simulink model "Model_Following_Approach"  (Simulink 7.5)
settings: Solver=ode45  StartTime=0.0  StopTime=10.0  RelTol=1e-3
values from neighbouring files (symbols this model uses):
  A_r = [ -1  -1   0   0 ... (first row only)    [main_c.m]    (also in main_elca.m; main_elca_nonsquare.m; main_elca_siso.m; main_elca_siso_conference.m)
  B_r = [ 1  0 ... (first row only)    [main_c.m]    (also in main_elca.m; main_elca_nonsquare.m = B_r(:,1:m); main_elca_siso.m = B_r(:,1:m); main_elca_siso_conference.m = [ 1)
  C_r = [ 1  0  0  0 ... (first row only)    [main_c.m]    (also in main_elca.m; main_elca_nonsquare.m = C_r(1:p,:); main_elca_siso.m = C_r(1:p,:); main_elca_siso_conference.m = [ 1  0  0  0])
  D_r = zeros(pr,mr)    [main_c.m]    (also in main_elca.m; main_elca_nonsquare.m; main_elca_siso.m; main_elca_siso_conference.m)
  Er = -inv(Rr)*B_r'*inv( A_r - B_r*Kr )'*C_r'*Qr    [main_c.m]    (also in main_elca.m; main_elca_nonsquare.m; main_elca_siso.m; main_elca_siso_conference.m)
  x_r = X_r'    [main_c.m]    (also in main_elca.m; main_elca_nonsquare.m; main_elca_siso.m; main_elca_siso_conference.m)
undefined symbols (not defined in the file or in its folder): Kr
settings Model: Creator=koni  LastModifiedBy=koni

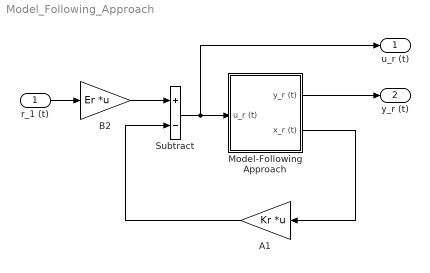
== system Model_Following_Approach ==
  r_1 (t) : Inport  PortDimensions=pr
  " Model-Following Approach" : Subsystem
  A1 : Gain  Gain=Kr  Multiplication=Matrix(K*u)  ParameterDataType=fixdt(1, 16)  ParameterScaling=2^0  OutDataType=fixdt(1, 16)  OutScaling=2^0
  B2 : Gain  Gain=Er  Multiplication=Matrix(K*u)  ParameterDataType=fixdt(1, 16)  ParameterScaling=2^0  OutDataType=fixdt(1, 16)  OutScaling=2^0
  Subtract : Sum  Inputs=+-  OutDataType=fixdt(1, 16)  OutScaling=2^-10
  u_r (t) : Outport  PortDimensions=mr  OutDataType=fixdt(1, 16)  OutScaling=2^0
  y_r (t) : Outport  Port=2  PortDimensions=pr  OutDataType=fixdt(1, 16)  OutScaling=2^0
  wires:
  " Model-Following Approach"/1(y_r (t)) -> y_r (t)/1
  Subtract/1 -> " Model-Following Approach"/1(u_r (t)), u_r (t)/1
  B2/1 -> Subtract/1
  r_1 (t)/1 -> B2/1
  " Model-Following Approach"/2(x_r (t)) -> A1/1
  A1/1 -> Subtract/2

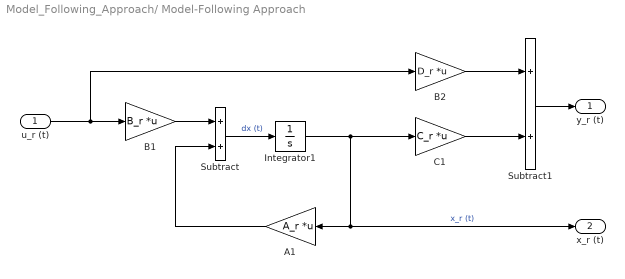
== system Model_Following_Approach/ Model-Following Approach ==
  u_r (t) : Inport  PortDimensions=mr
  A1 : Gain  Gain=A_r  Multiplication=Matrix(K*u)  ParameterDataType=fixdt(1, 16)  ParameterScaling=2^0  OutDataType=fixdt(1, 16)  OutScaling=2^0
  B1 : Gain  Gain=B_r  Multiplication=Matrix(K*u)  ParameterDataType=fixdt(1, 16)  ParameterScaling=2^0  OutDataType=fixdt(1, 16)  OutScaling=2^0
  B2 : Gain  Gain=D_r  Multiplication=Matrix(K*u)  ParameterDataType=fixdt(1, 16)  ParameterScaling=2^0  OutDataType=fixdt(1, 16)  OutScaling=2^0
  C1 : Gain  Gain=C_r  Multiplication=Matrix(K*u)  ParameterDataType=fixdt(1, 16)  ParameterScaling=2^0  OutDataType=fixdt(1, 16)  OutScaling=2^0
  Integrator1 : Integrator  InitialCondition=x_r(:,1)
  Subtract : Sum  OutDataType=fixdt(1, 16)  OutScaling=2^-10
  Subtract1 : Sum  OutDataType=fixdt(1, 16)  OutScaling=2^-10
  y_r (t) : Outport  PortDimensions=pr
  x_r (t) : Outport  Port=2  PortDimensions=nr
  wires:
  Subtract/1 -> Integrator1/1  "dx (t)"
  Integrator1/1 -> C1/1, A1/1, x_r (t)/1  "x_r (t)"
  u_r (t)/1 -> B1/1, B2/1
  B1/1 -> Subtract/1
  A1/1 -> Subtract/2
  Subtract1/1 -> y_r (t)/1
  C1/1 -> Subtract1/2
  B2/1 -> Subtract1/1
